simulink model "TunedGains"  (R2014a)
settings: Solver=ode45  StartTime=0.0  StopTime=10.0  RelTol=1e-3
libraries: simulink x2
settings Model: Creator=darenlee  LastModifiedBy=darenlee

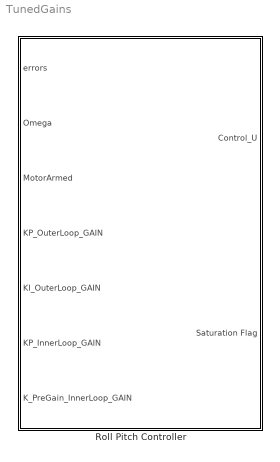
== system TunedGains ==
  Roll Pitch Controller : Subsystem  TreatAsAtomicUnit=on

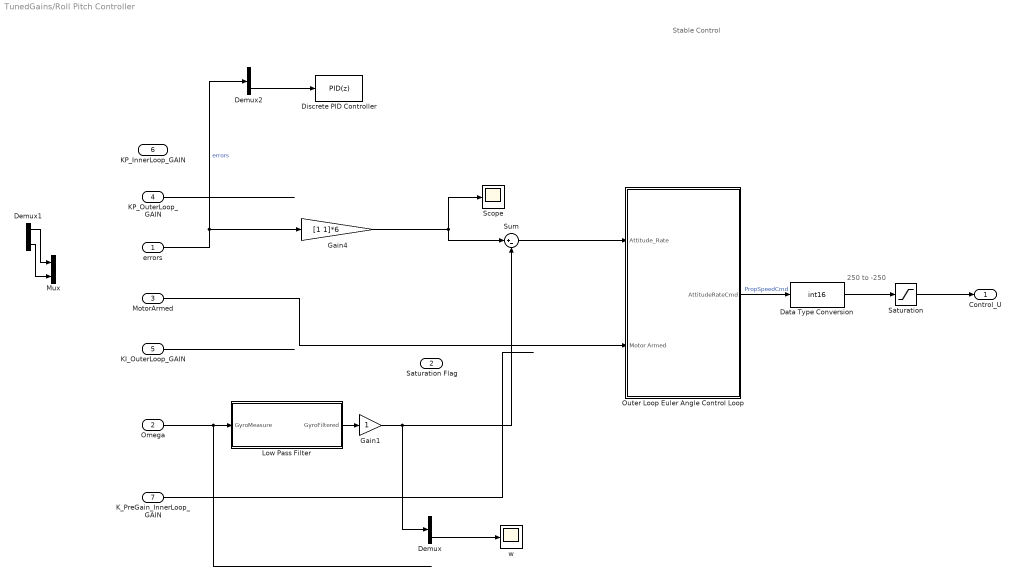
== system TunedGains/Roll Pitch Controller ==
  note: 250 to -250
  note: Stable Control
  errors : Inport
  Omega : Inport  Port=2
  MotorArmed : Inport  Port=3
  KP_OuterLoop_GAIN : Inport  Port=4
  KI_OuterLoop_GAIN : Inport  Port=5
  KP_InnerLoop_GAIN : Inport  Port=6
  K_PreGain_InnerLoop_GAIN : Inport  Port=7
  Data Type Conversion : DataTypeConversion  OutDataTypeStr=int16  RndMeth=Nearest
  Demux : Demux  Outputs=2
  Demux1 : Demux  Outputs=2
  Demux2 : Demux  Outputs=2
  Discrete PID Controller : simulink/Continuous/PID Controller  Controller=PID  TimeDomain=Discrete-time  SampleTime=-1  IntegratorMethod=Forward Euler  FilterMethod=Forward Euler  Form=Parallel  P=2.83495745743949  I=2.32367440623623  D=0.738560121288318*0  N=116.921248611606  InitialConditionSource=internal  InitialConditionForIntegrator=0  InitialConditionForFilter=0  ExternalReset=none  LimitOutput=on  UpperSaturationLimit=30  LowerSaturationLimit=-30  LinearizeAsGain=off  AntiWindupMode=back-calculation  Kb=1  TrackingMode=off  Kt=1  PParamMin=[]  PParamMax=[]  IParamMin=[]  IParamMax=[]  DParamMin=[]  DParamMax=[]  NParamMin=[]  NParamMax=[]  KbParamMin=[]  KbParamMax=[]  KtParamMin=[]  KtParamMax=[]  POutMin=[]  POutMax=[]  IOutMin=[]  IOutMax=[]  DOutMin=[]  DOutMax=[]  NOutMin=[]  NOutMax=[]  KbOutMin=[]  KbOutMax=[]  KtOutMin=[]  KtOutMax=[]  IntegratorOutMin=[]  IntegratorOutMax=[]  FilterOutMin=[]  FilterOutMax=[]  SumOutMin=[]  SumOutMax=[]  SumI1OutMin=[]  SumI1OutMax=[]  SumI2OutMin=[]  SumI2OutMax=[]  SumI3OutMin=[]  SumI3OutMax=[]  SumDOutMin=[]  SumDOutMax=[]  SaturationOutMin=[]  SaturationOutMax=[]  IntegratorContinuousStateAttributes=''  IntegratorStateMustResolveToSignalObject=off  IntegratorRTWStateStorageClass=Auto  FilterContinuousStateAttributes=''  FilterStateMustResolveToSignalObject=off  FilterRTWStateStorageClass=Auto
  Gain1 : Gain
  Gain4 : Gain  Gain=[1 1]*6
  Low Pass Filter : Subsystem
  Mux : Mux  Inputs=2
  Outer Loop Euler Angle Control Loop : Subsystem
  Saturation : Saturate  UpperLimit=250  LowerLimit=-250  OutDataTypeStr=int16
      settings: AttributesFormatString=%<LowerLimit>\nto\n%<UpperLimit>
  Scope : Scope
      settings: SaveName=SwitchSignal_Attitude_Rate
  Sum : Sum  Inputs=|+-
  w : Scope
      settings: YMin=-45  YMax=55  SaveName=ScopeData16
  Control_U : Outport
  Saturation Flag : Outport  Port=2
  wires:
  Saturation/1 -> Control_U/1
  Data Type Conversion/1 -> Saturation/1
  K_PreGain_InnerLoop_GAIN/1 -> ?
  Outer Loop Euler Angle Control Loop/1(AttitudeRateCmd) -> Data Type Conversion/1  "PropSpeedCmd"
  KP_OuterLoop_GAIN/1 -> ?
  MotorArmed/1 -> Outer Loop Euler Angle Control Loop/2(Motor Armed)
  KI_OuterLoop_GAIN/1 -> ?
  ? -> Saturation Flag/1
  Omega/1 -> Low Pass Filter/1(GyroMeasure)
  errors/1 -> Gain4/1, Demux2/1  "errors"
  ? -> Demux1/1
  Demux1/1 -> Mux/1
  Demux2/2 -> Discrete PID Controller/1
  Demux1/2 -> Mux/2
  Demux/2 -> w/1
  Low Pass Filter/1(GyroFiltered) -> Gain1/1
  Sum/1 -> Outer Loop Euler Angle Control Loop/1(Attitude_Rate)
  Gain4/1 -> Sum/1, Scope/1
  Gain1/1 -> Sum/2, Demux/1

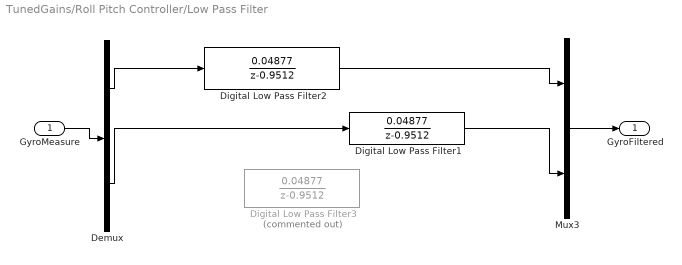
== system TunedGains/Roll Pitch Controller/Low Pass Filter ==
  GyroMeasure : Inport
  Demux : Demux  Outputs=2
  Digital Low Pass Filter1 : DiscreteTransferFcn  Numerator=[0.04877]  Denominator=[1 -0.9512]  OutDataTypeStr=int16
  Digital Low Pass Filter2 : DiscreteTransferFcn  Numerator=[0.04877]  Denominator=[1 -0.9512]  OutDataTypeStr=int16
  Digital Low Pass Filter3 : DiscreteTransferFcn  Commented=on  Numerator=[0.04877]  Denominator=[1 -0.9512]  OutDataTypeStr=int16
  Mux3 : Mux  Inputs=2
  GyroFiltered : Outport
  wires:
  Mux3/1 -> GyroFiltered/1
  Demux/1 -> Digital Low Pass Filter2/1
  GyroMeasure/1 -> Demux/1
  Demux/2 -> Digital Low Pass Filter1/1
  Digital Low Pass Filter2/1 -> Mux3/1
  Digital Low Pass Filter1/1 -> Mux3/2

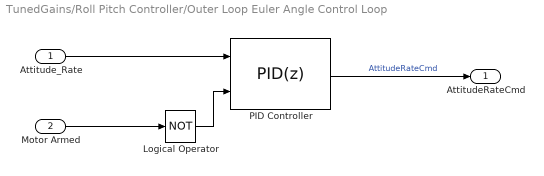
== system TunedGains/Roll Pitch Controller/Outer Loop Euler Angle Control Loop ==
  Attitude_Rate : Inport
  Motor Armed : Inport  Port=2
  Logical Operator : Logic  Operator=NOT  AllPortsSameDT=off  OutDataTypeStr=boolean
  PID Controller : simulink/Continuous/PID Controller  Controller=PID  TimeDomain=Discrete-time  SampleTime=-1  IntegratorMethod=Forward Euler  FilterMethod=Forward Euler  Form=Parallel  P=0.10084  I=0.13631  D=-0.011755  N=5  InitialConditionSource=internal  InitialConditionForIntegrator=0  InitialConditionForFilter=0  ExternalReset=level  LimitOutput=on  UpperSaturationLimit=30  LowerSaturationLimit=-30  LinearizeAsGain=on  AntiWindupMode=clamping  Kb=1  TrackingMode=off  Kt=1  PParamMin=[]  PParamMax=[]  IParamMin=[]  IParamMax=[]  DParamMin=[]  DParamMax=[]  NParamMin=[]  NParamMax=[]  KbParamMin=[]  KbParamMax=[]  KtParamMin=[]  KtParamMax=[]  POutMin=[]  POutMax=[]  IOutMin=[]  IOutMax=[]  DOutMin=[]  DOutMax=[]  NOutMin=[]  NOutMax=[]  KbOutMin=[]  KbOutMax=[]  KtOutMin=[]  KtOutMax=[]  IntegratorOutMin=[]  IntegratorOutMax=[]  FilterOutMin=[]  FilterOutMax=[]  SumOutMin=[]  SumOutMax=[]  SumI1OutMin=[]  SumI1OutMax=[]  SumI2OutMin=[]  SumI2OutMax=[]  SumI3OutMin=[]  SumI3OutMax=[]  SumDOutMin=[]  SumDOutMax=[]  SaturationOutMin=[]  SaturationOutMax=[]  IntegratorContinuousStateAttributes=''  IntegratorStateMustResolveToSignalObject=off  IntegratorRTWStateStorageClass=Auto  FilterContinuousStateAttributes=''  FilterStateMustResolveToSignalObject=off  FilterRTWStateStorageClass=Auto
  AttitudeRateCmd : Outport
  wires:
  PID Controller/1 -> AttitudeRateCmd/1  "AttitudeRateCmd"
  Motor Armed/1 -> Logical Operator/1
  Logical Operator/1 -> PID Controller/2
  Attitude_Rate/1 -> PID Controller/1
